simulink model "test_induction_cooker_potremovedwhilecooking"  (R2022b)
settings: Solver=FixedStepAuto  StartTime=0.0  StopTime=120  FixedStep=0.1  RelTol=1e-3
settings Model: Creator=alewi  LastModifiedBy=cristian
settings ConfigComp: CovEnable=on  CovScope=ReferencedModels  CovIncludeTopModel=off  CovModelRefEnable=filtered

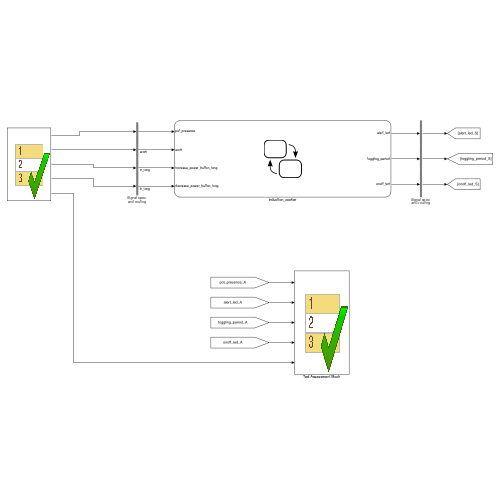
[thumbnail: Simulink's stored preview of the top-level diagram]
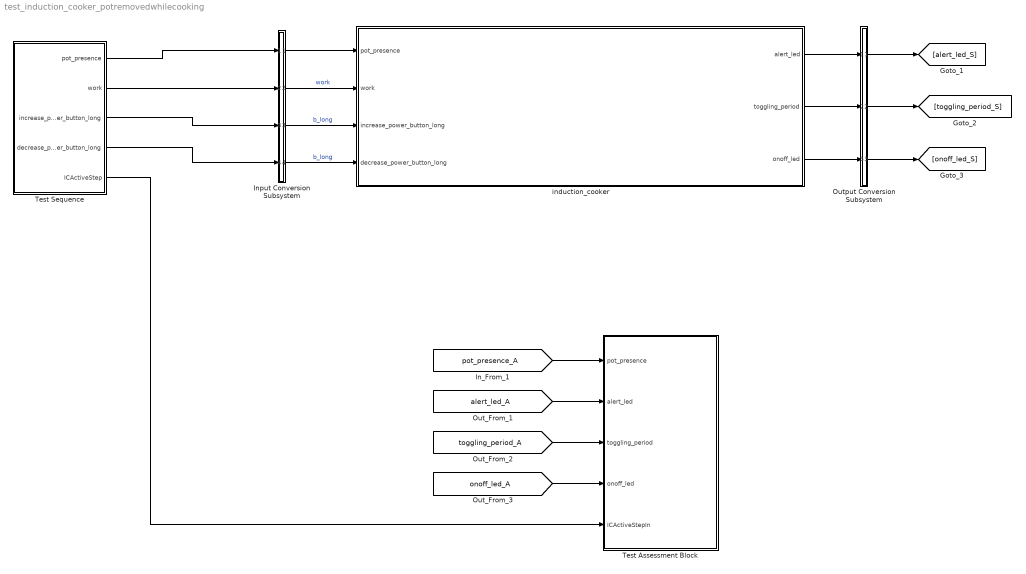
== system test_induction_cooker_potremovedwhilecooking ==
  Input Conversion Subsystem : Subsystem  Tag=__SLT_ICS__  Description=|
      | Signal spec.
      | and routing
      settings: AttributesFormatString=%<Description>
  Output Conversion Subsystem : Subsystem  Tag=__SLT_OCS__  Description=|
      | Signal spec.
      | and routing
      settings: AttributesFormatString=%<Description>
  Test Assessment Block : Test Sequence  Tag=__SLT_ASMT__  TreatAsAtomicUnit=on
  Test Sequence : Test Sequence  TreatAsAtomicUnit=on
  induction_cooker : Stateflow chart  TreatAsAtomicUnit=on
  wires:
  Test Sequence/1(pot_presence) -> Input Conversion Subsystem/1(Inport_1)
  Test Sequence/2(work) -> Input Conversion Subsystem/2(Inport_2)
  Test Sequence/3(increase_power_button_long) -> Input Conversion Subsystem/3(Inport_3)
  Test Sequence/4(decrease_power_button_long) -> Input Conversion Subsystem/4(Inport_4)
  Output Conversion Subsystem/1(Outport_1) -> [alert_led_S]
  Output Conversion Subsystem/2(Outport_2) -> [toggling_period_S]
  Output Conversion Subsystem/3(Outport_3) -> [onoff_led_S]
  Input Conversion Subsystem/1(Outport_1) -> induction_cooker/1(pot_presence)
  Input Conversion Subsystem/2(Outport_2) -> induction_cooker/2(work)  "work"
  Input Conversion Subsystem/3(Outport_3) -> induction_cooker/3(increase_power_button_long)  "b_long"
  Input Conversion Subsystem/4(Outport_4) -> induction_cooker/4(decrease_power_button_long)  "b_long"
  induction_cooker/1(alert_led) -> Output Conversion Subsystem/1(Inport_1)
  induction_cooker/2(toggling_period) -> Output Conversion Subsystem/2(Inport_2)
  induction_cooker/3(onoff_led) -> Output Conversion Subsystem/3(Inport_3)
  [onoff_led_A] -> Test Assessment Block/4(onoff_led)
  Test Sequence/5(ICActiveStep) -> Test Assessment Block/5(ICActiveStepIn)
  [toggling_period_A] -> Test Assessment Block/3(toggling_period)
  [alert_led_A] -> Test Assessment Block/2(alert_led)
  [pot_presence_A] -> Test Assessment Block/1(pot_presence)

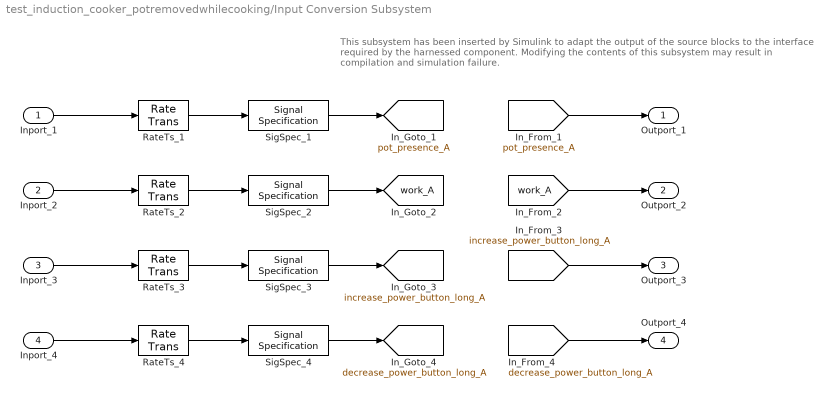
== system test_induction_cooker_potremovedwhilecooking/Input Conversion Subsystem ==
  note: This subsystem has been inserted by Simulink to adapt the output of the source blocks to the interface required by the harnessed component.
      |  Modifying the contents of this subsystem may result in compilation and simulation failure.
  Inport_1 : Inport
  Inport_2 : Inport  Port=2
  Inport_3 : Inport  Port=3
  Inport_4 : Inport  Port=4
  RateTs_1 : RateTransition  OutPortSampleTime=[-1, 0]
  RateTs_2 : RateTransition  OutPortSampleTime=[0, 1]
  RateTs_3 : RateTransition  OutPortSampleTime=[0, 1]
  RateTs_4 : RateTransition  OutPortSampleTime=[0, 1]
  SigSpec_1 : SignalSpecification  OutDataTypeStr=boolean  Dimensions=[1]  SampleTime=[-1, 0]
  SigSpec_2 : SignalSpecification  OutDataTypeStr=boolean  Dimensions=[1]  SampleTime=[0, 1]
  SigSpec_3 : SignalSpecification  OutDataTypeStr=boolean  Dimensions=[1]  SampleTime=[0, 1]
  SigSpec_4 : SignalSpecification  OutDataTypeStr=boolean  Dimensions=[1]  SampleTime=[0, 1]
  Outport_1 : Outport
  Outport_2 : Outport  Port=2
  Outport_3 : Outport  Port=3
  Outport_4 : Outport  Port=4
  tag scope: decrease_power_button_long_A=global, increase_power_button_long_A=global, pot_presence_A=global, work_A=global
  wires:
  [pot_presence_A] -> Outport_1/1
  SigSpec_1/1 -> [pot_presence_A]
  RateTs_1/1 -> SigSpec_1/1
  Inport_1/1 -> RateTs_1/1
  [work_A] -> Outport_2/1
  SigSpec_2/1 -> [work_A]
  RateTs_2/1 -> SigSpec_2/1
  Inport_2/1 -> RateTs_2/1
  [increase_power_button_long_A] -> Outport_3/1
  SigSpec_3/1 -> [increase_power_button_long_A]
  RateTs_3/1 -> SigSpec_3/1
  Inport_3/1 -> RateTs_3/1
  [decrease_power_button_long_A] -> Outport_4/1
  SigSpec_4/1 -> [decrease_power_button_long_A]
  RateTs_4/1 -> SigSpec_4/1
  Inport_4/1 -> RateTs_4/1

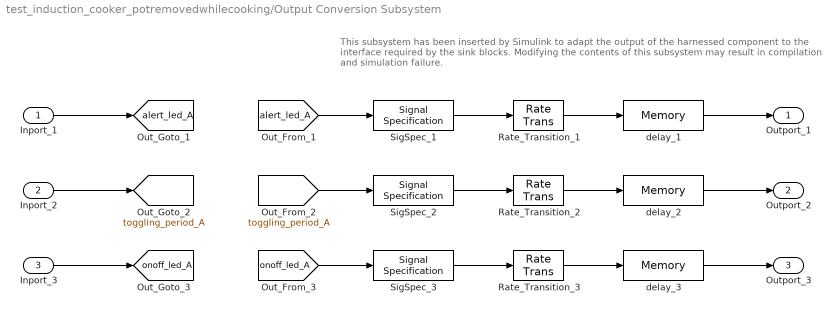
== system test_induction_cooker_potremovedwhilecooking/Output Conversion Subsystem ==
  note: This subsystem has been inserted by Simulink to adapt the output of the harnessed component to the interface required by the sink blocks.
      |  Modifying the contents of this subsystem may result in compilation and simulation failure.
  Inport_1 : Inport
  Inport_2 : Inport  Port=2
  Inport_3 : Inport  Port=3
  Rate_Transition_1 : RateTransition  OutPortSampleTimeOpt=Inherit
  Rate_Transition_2 : RateTransition  OutPortSampleTimeOpt=Inherit
  Rate_Transition_3 : RateTransition  OutPortSampleTimeOpt=Inherit
  SigSpec_1 : SignalSpecification  OutDataTypeStr=boolean  Dimensions=[1]
  SigSpec_2 : SignalSpecification  OutDataTypeStr=double  Dimensions=[1]
  SigSpec_3 : SignalSpecification  OutDataTypeStr=boolean  Dimensions=[1]
  delay_1 : Memory
  delay_2 : Memory
  delay_3 : Memory
  Outport_1 : Outport
  Outport_2 : Outport  Port=2
  Outport_3 : Outport  Port=3
  tag scope: alert_led_A=global, onoff_led_A=global, toggling_period_A=global
  wires:
  Inport_1/1 -> [alert_led_A]
  [alert_led_A] -> SigSpec_1/1
  SigSpec_1/1 -> Rate_Transition_1/1
  Rate_Transition_1/1 -> delay_1/1
  delay_1/1 -> Outport_1/1
  Inport_2/1 -> [toggling_period_A]
  [toggling_period_A] -> SigSpec_2/1
  SigSpec_2/1 -> Rate_Transition_2/1
  Rate_Transition_2/1 -> delay_2/1
  delay_2/1 -> Outport_2/1
  Inport_3/1 -> [onoff_led_A]
  [onoff_led_A] -> SigSpec_3/1
  SigSpec_3/1 -> Rate_Transition_3/1
  Rate_Transition_3/1 -> delay_3/1
  delay_3/1 -> Outport_3/1

== stateflow chart test_induction_cooker_potremovedwhilecooking/Test Assessment Block ==
  state PotRemovedWhileCooking
    state step_1
      state VerifyPotRemovedWhileCooking_Init
        verify(pot_presence == 0 && alert_led == 0 && abs(toggling_period - 0) < TOLERANCE && onoff_led == 0)
        settings: description=Si controlla lo stato inziale della macchina.
      state VerifyPotRemovedWhileCooking_PowerOn
        verify(pot_presence == 0 && alert_led == 0 && abs(toggling_period - 0) < TOLERANCE && onoff_led == 1)
        settings: description=La macchina è accesa: solo il led di accensione deve risultare attivo.
      state VerifyPotRemovedWhileCooking_PressFor300W
        verify(pot_presence == 0 && alert_led == 0 && abs(toggling_period - 0) < TOLERANCE && onoff_led == 1)
        settings: description=|
            | Il pulsante di incremento potenza è stato appena premuto.
            | Lo stato dei led e delle variabili interne deve rimanere inalterato.
      state VerifyPotRemovedWhileCooking_ReleaseFor300W
        verify(pot_presence == 0 && alert_led == 0 && abs(toggling_period - 0) < TOLERANCE && onoff_led == 1)
        settings: description=|
            | Il pulsante è stato rilasciato.
            | Lo stato dei led e delle variabili interne deve rimanere inalterato.
      state VerifyPotRemovedWhileCooking_WaitIn300W
        verify(pot_presence == 0 && alert_led == 0 && abs(toggling_period - 2) < TOLERANCE && onoff_led == 1)
        settings: description=|
            | La potenza viene effettivamente cambiata.
            | Essendo la macchina nello stato dei 300W, il periodo di blinking deve essere di 2 secondi.
      state VerifyIncreaseDecreasePower_RemovePot
        verify(pot_presence == 1 && alert_led == 1 && abs(toggling_period - 2) < TOLERANCE && onoff_led == 1)
        settings: description=|
            | La pentola viene rimossa.
            | Lo stato del led di alert deve essere attivo.
      state VerifyIncreaseDecreasePower_ResetState
        verify(pot_presence == 1 && alert_led == 0 && abs(toggling_period - 0) < TOLERANCE && onoff_led == 1)
        settings: description=|
            | Il timeout per attendere che la pentola venga riposizionata è scaduto.
            | La macchina viene resettata.
            | Il periodo di blinking è tornato a 0 secondi.
            | Il led di alert viene spento.
      state step_1_1
      step_1 -> (junction 498)
      (default) -> (junction 498)
      (junction 498) -> (junction 499) [order 1] : [ICActiveStepIn == ICActiveStepEnum.PotRemovedWhileCooking_Init
          | ]
      (junction 499) -> VerifyPotRemovedWhileCooking_Init [order 1] : [~in(PotRemovedWhileCooking.step_1.VerifyPotRemovedWhileCooking_Init)]
      (junction 498) -> (junction 509) [order 2]
      (junction 499) -> (junction 502) [order 2]
      (junction 509) -> (junction 510) [order 1] : [ICActiveStepIn == ICActiveStepEnum.PotRemovedWhileCooking_PowerOn
          | ]
      (junction 510) -> VerifyPotRemovedWhileCooking_PowerOn [order 1] : [~in(PotRemovedWhileCooking.step_1.VerifyPotRemovedWhileCooking_PowerOn)]
      (junction 509) -> (junction 517) [order 2]
      (junction 510) -> (junction 513) [order 2]
      (junction 517) -> (junction 518) [order 1] : [ICActiveStepIn == ICActiveStepEnum.PotRemovedWhileCooking_PressFor300W
          | ]
      (junction 518) -> VerifyPotRemovedWhileCooking_PressFor300W [order 1] : [~in(PotRemovedWhileCooking.step_1.VerifyPotRemovedWhileCooking_PressFor300W)]
      (junction 517) -> (junction 525) [order 2]
      (junction 518) -> (junction 521) [order 2]
      (junction 525) -> (junction 526) [order 1] : [ICActiveStepIn == ICActiveStepEnum.PotRemovedWhileCooking_ReleaseFor300W
          | ]
      (junction 526) -> VerifyPotRemovedWhileCooking_ReleaseFor300W [order 1] : [~in(PotRemovedWhileCooking.step_1.VerifyPotRemovedWhileCooking_ReleaseFor300W)]
      (junction 525) -> (junction 533) [order 2]
      (junction 526) -> (junction 529) [order 2]
      (junction 533) -> (junction 534) [order 1] : [ICActiveStepIn == ICActiveStepEnum.PotRemovedWhileCooking_WaitIn300W
          | ]
      (junction 534) -> VerifyPotRemovedWhileCooking_WaitIn300W [order 1] : [~in(PotRemovedWhileCooking.step_1.VerifyPotRemovedWhileCooking_WaitIn300W)]
      (junction 533) -> (junction 541) [order 2]
      (junction 534) -> (junction 537) [order 2]
      (junction 541) -> (junction 542) [order 1] : [ICActiveStepIn == ICActiveStepEnum.PotRemovedWhileCooking_RemovePot
          | ]
      (junction 542) -> VerifyIncreaseDecreasePower_RemovePot [order 1] : [~in(PotRemovedWhileCooking.step_1.VerifyIncreaseDecreasePower_RemovePot)]
      (junction 541) -> (junction 549) [order 2]
      (junction 542) -> (junction 545) [order 2]
      (junction 549) -> (junction 550) [order 1] : [ICActiveStepIn == ICActiveStepEnum.PotRemovedWhileCooking_ResetState
          | ]
      (junction 550) -> VerifyIncreaseDecreasePower_ResetState [order 1] : [~in(PotRemovedWhileCooking.step_1.VerifyIncreaseDecreasePower_ResetState)]
      (junction 550) -> (junction 553) [order 2]
      (junction 557) -> (junction 558)
      (junction 558) -> step_1_1 [order 1] : [~in(PotRemovedWhileCooking.step_1.step_1_1)]
      (junction 558) -> (junction 561) [order 2]
      (junction 549) -> (junction 557) [order 2]
    (default) -> step_1
  (default) -> PotRemovedWhileCooking : {assert(Active_Scenario_Index == 1,'The value of Scenario Parameter ''Active_Scenario_Index'' is not valid. Use the index of the scenario to specify it.')}
  data: pot_presence input boolean size=[1]; alert_led input boolean size=[1]; toggling_period input double size=[1]; onoff_led input boolean size=[1]; ICActiveStepIn input; Active_Scenario_Index parameter =1; TOLERANCE constant double =1e-9; sample_time constant double =str2num(get_param('InductionCooker','FixedStep'))

== stateflow chart test_induction_cooker_potremovedwhilecooking/induction_cooker ==
  note: Il core del fornello è composto da un chart principale che oscilla tra uno stato ON ed uno stato OFF, a seconda dell'input work che ne indica in che stato di funzionamento deve essere (associato al bottone a livelli di on/off).
  state OFF
    en: onoff_led = LOW, alert_led = LOW,
    current_power = 0, toggling_period = TOGGLING_PERIOD_OFF
  note: Lo stato ON è composto da tre macchine parallele che gestiscono rispettivamente: cambiamento potenza, allarme e blink del led.
  state ON
    state LOGIC [parallel]
      settings: executionOrder=1
      note: In LOGIC, lo stato di ingresso è quello a 0W, in quanto appena accendiamo il fornello esso non è attivo.
          | Quando si riceve l'input di INCREASE o DECREASE button, si transita in uno stato che rappresenta una nuova potenza selezionata, dopo 5 secondi da un passaggio di stato la potenza reale diventerà quella associata allo stato correntemente attivo.
          | Quando una certa potenza viene selezionata, viene aggiornato il periodo di blink del power_led.
      state P0W
        state WAIT
        state SET
          en:
          current_power = 0, toggling_period = TOGGLING_PERIOD_0W
        note: Lo stato che rappresenta 0W gode della particolarità di poter fissare la potenza anche senza attendere i 5s, questo è possibile quando da uno stato gerarchicamente superiore o parallelo viene impostato current_power = 0W. Tale circostanza avviene sia all'avvio in cui non vi è necessità di attendere del tempo prima di impostare la potenza a 0W e sia nel momento in cui scatta l'allarme, in cui si disattiva il fornello istantaneamente.
        (default) -> ON.LOGIC.P0W.WAIT
        ON.LOGIC.P0W.WAIT -> ON.LOGIC.P0W.SET : [after(SET_POWER_PATIENCE,sec) || current_power == 0]
      note: Notiamo che in ogni stato di LOGIC, diverso da 0W, vi è una transizione associata al fatto che la variabile alarm assume valore HIGH, che ci riporta automaticamente nello stato 0W e fissa tale potenza come potenza corrente senza attendere i 10 secondi.
      state P1500W
        state WAIT
        state SET
          en:
          current_power = 1500, toggling_period = TOGGLING_PERIOD_1500W
        (default) -> ON.LOGIC.P1500W.WAIT
        ON.LOGIC.P1500W.WAIT -> ON.LOGIC.P1500W.SET : after(SET_POWER_PATIENCE,sec)
      state P300W
        state WAIT
        state SET
          en:
          current_power = 300, toggling_period = TOGGLING_PERIOD_300W
        (default) -> ON.LOGIC.P300W.WAIT
        ON.LOGIC.P300W.WAIT -> ON.LOGIC.P300W.SET : after(SET_POWER_PATIENCE,sec)
      state P1000W
        state WAIT
        state SET
          en:
          current_power = 1000, toggling_period = TOGGLING_PERIOD_1000W
        (default) -> ON.LOGIC.P1000W.WAIT
        ON.LOGIC.P1000W.WAIT -> ON.LOGIC.P1000W.SET : after(SET_POWER_PATIENCE,sec)
      state P500W
        state WAIT
        state SET
          en:
          current_power = 500, toggling_period = TOGGLING_PERIOD_500W
        (default) -> ON.LOGIC.P500W.WAIT
        ON.LOGIC.P500W.WAIT -> ON.LOGIC.P500W.SET : after(SET_POWER_PATIENCE,sec)
      (default) -> P0W
      P1500W -> P0W [order 2] : [alarm == HIGH]
      P0W -> P300W : [increase_power_button_long == PRESSED && pot_presence == PRESSED]
      P300W -> P0W [order 1] : [(alarm == HIGH) || (decrease_power_button_long == PRESSED && pot_presence == PRESSED)]
      P500W -> P0W [order 3] : [alarm == HIGH]
      P1000W -> P0W [order 3] : [alarm == HIGH]
      P500W -> P300W [order 1] : [decrease_power_button_long == PRESSED && pot_presence == PRESSED]
      P300W -> P500W [order 2] : [increase_power_button_long == PRESSED && pot_presence == PRESSED]
      P1500W -> P1000W [order 1] : [decrease_power_button_long == PRESSED && pot_presence == PRESSED]
      P1000W -> P1500W [order 2] : [increase_power_button_long == PRESSED && pot_presence == PRESSED]
      P500W -> P1000W [order 2] : [increase_power_button_long == PRESSED && pot_presence == PRESSED]
      P1000W -> P500W [order 1] : [decrease_power_button_long == PRESSED && pot_presence == PRESSED]
    state ALARM [parallel]
      settings: executionOrder=2
      state ACTIVE
        state QUIET
          en: alarm = LOW, alert_led = LOW
        state ALARM
          en: alert_led = HIGH
          on after(ALARM_PATIENCE,sec): alarm = HIGH; current_power = 0; toggling_period = TOGGLING_PERIOD_0W; alert_led = LOW;
        (default) -> QUIET
        QUIET -> ON.ALARM.ACTIVE.ALARM : [pot_presence == RELEASED]
        ON.ALARM.ACTIVE.ALARM -> QUIET : [pot_presence == PRESSED]
      state INACTIVE
        en:
        alarm = LOW,
        alert_led = LOW
      (default) -> INACTIVE
      INACTIVE -> ACTIVE : [current_power ~= 0]
      ACTIVE -> INACTIVE : [current_power == 0]
    state TOGGLING_LED [parallel] [commented out]
      note: In ogni stato di LOGIC, che rappresenta una specifica potenza, viene impostato un valore di periodo che indica ogni quanto il power_led (led giallo) lampeggia.
          | Infatti, tale macchina semplicemente rimbalza da uno stato all'altro accendendo e spegnendo il led.
      state LED_OFF [commented out]
        en: power_led=LOW;
      state LED_ON [commented out]
        en: power_led=HIGH;
      (default) -> LED_OFF [commented out]
      LED_OFF -> LED_ON [commented out] : [toggling_period>0 && after(toggling_period,sec)]
      LED_ON -> LED_OFF [commented out] : [after(toggling_period,sec)]
  note: Quando la macchina non è attiva (current_power = 0W), anche l'allarme è inattivo. All'attivazione del fornello corrisponde l'attivazione dell'allarme.
      | Nel momento in cui l'allarme è attivo e rileva una rimozione della pentola passa in uno stato ALARM che accende l'alert_led e dopo 10 secondi di permanenza disattiva il sistema portando LOGIC nello stato 0W, a meno di reinserimento pentola che riporta in uno stato QUIET.
  (default) -> OFF
  OFF -> ON : [work == HIGH]{onoff_led = HIGH}
  ON -> OFF : [work == LOW]
  data: pot_presence input boolean size=1; work input boolean size=1; alarm local boolean size=1; alert_led output boolean size=1; toggling_period output double size=1; onoff_led output boolean size=1; current_power local uint16 size=1; increase_power_button_long input boolean size=1; decrease_power_button_long input boolean size=1; HIGH constant boolean size=1 =1; PRESSED constant boolean size=1 =0; RELEASED constant boolean size=1 =1; LOW constant boolean size=1 =0; ALARM_PATIENCE constant double =10; TOGGLING_PERIOD_0W constant double =0; TOGGLING_PERIOD_300W constant double =2; TOGGLING_PERIOD_500W constant double =1; TOGGLING_PERIOD_1000W constant double =0.5; TOGGLING_PERIOD_1500W constant double =0.25; SET_POWER_PATIENCE local =5; TOGGLING_PERIOD_OFF constant double =0

== stateflow chart test_induction_cooker_potremovedwhilecooking/Test Sequence ==
  settings: updateMethod=DISCRETE  sampleTime=0.1
  state PotRemovedWhileCooking
    state PotRemovedWhileCooking_Init
      pot_presence = false;
      work = false;
      increase_power_button_long = true;
      decrease_power_button_long = true;
      settings: description=|
          | La macchina è inizializzata.
          | La pentola è presente sul fornello.
    state PotRemovedWhileCooking_PowerOn
      work = true;
      settings: description=La macchina viene accesa.
    state PotRemovedWhileCooking_PressFor300W
      increase_power_button_long = false;
      settings: description=Viene premuto il pulsante per incrementare la potenza.
    state PotRemovedWhileCooking_ReleaseFor300W
      increase_power_button_long = true;
      settings: description=VIene rilasciato il pulsante per incrementare la potenza
    state PotRemovedWhileCooking_WaitIn300W
      settings: description=Si rimane a 300W per 3 secondi
    state PotRemovedWhileCooking_RemovePot
      pot_presence = true;
      settings: description=Viene rimosssa la pentola.
    state PotRemovedWhileCooking_ResetState
      settings: description=Sono stati attesi 10 secondi affinché la macchina venga resettata.
    (default) -> PotRemovedWhileCooking_Init
    PotRemovedWhileCooking_Init -> PotRemovedWhileCooking_PowerOn
    PotRemovedWhileCooking_PowerOn -> PotRemovedWhileCooking_PressFor300W : [
        | after(sample_time*2,sec)
        | ]
    PotRemovedWhileCooking_PressFor300W -> PotRemovedWhileCooking_ReleaseFor300W : [
        | true
        | ]
    PotRemovedWhileCooking_ReleaseFor300W -> PotRemovedWhileCooking_WaitIn300W : [
        | after(5-sample_time,sec)
        | ]
    PotRemovedWhileCooking_WaitIn300W -> PotRemovedWhileCooking_RemovePot : [
        | after(3,sec)
        | ]
    PotRemovedWhileCooking_RemovePot -> PotRemovedWhileCooking_ResetState : [
        | after(10,sec)
        | ]
  (default) -> PotRemovedWhileCooking : {assert(Active_Scenario_Index == 1,'The value of Scenario Parameter ''Active_Scenario_Index'' is not valid. Use the index of the scenario to specify it.')}
  data: pot_presence output boolean size=[1]; work output boolean size=[1]; increase_power_button_long output boolean size=[1]; decrease_power_button_long output boolean size=[1]; ICActiveStep output Enum: ICActiveStepEnum; Active_Scenario_Index parameter =1; sample_time constant double =str2num(get_param('InductionCooker','FixedStep'))
